simulink model "HILSimulation"  (R2021a)
settings: Solver=FixedStepAuto  StartTime=0.0  StopTime=Inf  FixedStep=sample_time  RelTol=1e-3
InitFcn:
  | SampleTime
values from neighbouring files (symbols this model uses):
  sample_time = 0.05    [SampleTime.m]
undefined symbols (not defined in the file or in its folder): LF
libraries: instrumentseriallib x3, slrealtimeutilitieslib x1
settings Model: EnablePacing=on  Creator=computador  LastModifiedBy=computador

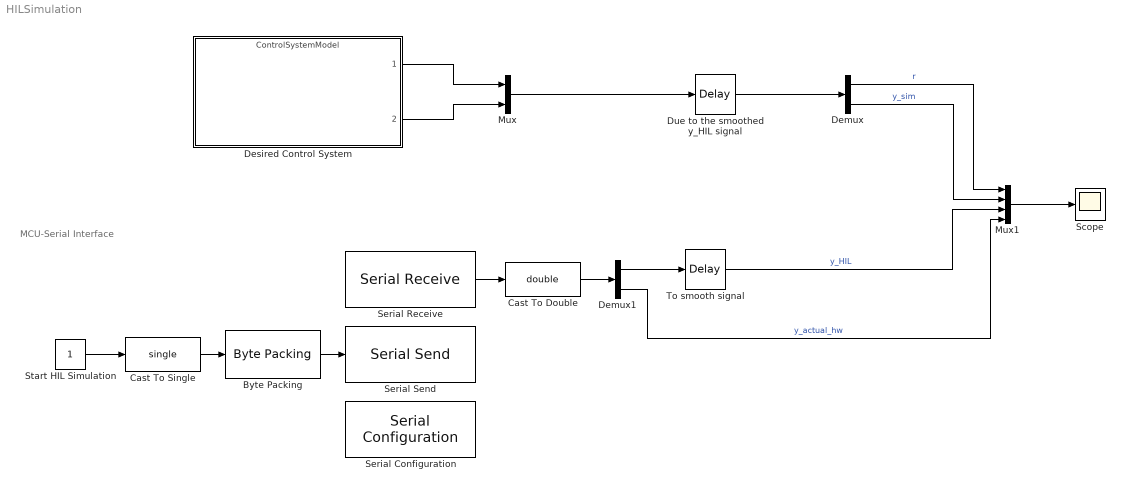
== system HILSimulation ==
  note: MCU-Serial Interface
  Byte Packing : slrealtimeutilitieslib/Byte Packing  MaskPackedDataType=uint32  MaskUnpackedDataTypes={'single'}  MaskAlignment=4
  Cast To Double : DataTypeConversion  OutDataTypeStr=double
  Cast To Single : DataTypeConversion  OutDataTypeStr=single
  Demux : Demux  Outputs=2
  Demux1 : Demux  Outputs=2
  Desired Control System : ModelReference  ModelNameDialog=ControlSystemModel.slx  SimulationMode=Normal  ModelReferenceVersion=1.12
  Due to the smoothed y_HIL signal : TransportDelay  DelayTime=sample_time
  Mux : Mux  Inputs=2
  Mux1 : Mux
  Scope : Scope
  Serial Configuration : instrumentseriallib/Serial Configuration  Priority=-200000  Port=COM2  ComPort=COM2  BaudRate=115200  DataBits=8  Parity=none  StopBits=1  ByteOrder=little-endian  FlowControl=none  Timeout=10  SimulateUsing=Interpreted execution  BlockInModel=on
  Serial Receive : instrumentseriallib/Serial Receive  Priority=1  Port=COM2  ComPort=COM2  DataType=single  SaveDataType=uint8  ToggleHeader=on  Header='S'  ToggleTerminator=on  Terminator=LF ('\n')  CustomTerminator=[]  ToggleDataSize=on  DataSize=[1 2]  EnableBlockingMode=on  ActionDataUnavailable=Output last received value  ActionWhenDataUnavailable=Output last received value  CustomValue=0  SampleTime=sample_time  SimulateUsing=Interpreted execution  BlockInModel=on
  Serial Send : instrumentseriallib/Serial Send  Priority=1  Port=COM2  ComPort=COM2  Header=[]  Terminator=<none>  CustomTerminator=[]  EnableBlockingMode=on  SimulateUsing=Interpreted execution  BlockInModel=on
  Start HIL Simulation : Constant
  To smooth signal : TransportDelay  DelayTime=sample_time
  wires:
  Cast To Single/1 -> Byte Packing/1
  Byte Packing/1 -> Serial Send/1
  Start HIL Simulation/1 -> Cast To Single/1
  Serial Receive/1 -> Cast To Double/1
  Mux/1 -> Due to the smoothed y_HIL signal/1
  Desired Control System/1 -> Mux/1
  Desired Control System/2 -> Mux/2
  Due to the smoothed y_HIL signal/1 -> Demux/1
  Demux/1 -> Mux1/1  "r"
  Demux/2 -> Mux1/2  "y_sim"
  Cast To Double/1 -> Demux1/1
  Demux1/1 -> To smooth signal/1
  To smooth signal/1 -> Mux1/3  "y_HIL"
  Demux1/2 -> Mux1/4  "y_actual_hw"
  Mux1/1 -> Scope/1
